simulink model "Test"  (R2018b)
settings: Solver=VariableStepAuto  StartTime=0.0  StopTime=10.0  RelTol=1e-3
undefined symbols (not defined in the file or in its folder): ExpectedOutputs, Inputs, sigbuilder_block, TestCase, TestInps, TestIters
libraries: fillib x3, library x2
(part 3 of 7)

== stateflow chart Test/ XOR ==
  settings: stateMachineType=SIMPLIFIED_MACHINE
  state Init
    fb_select = 1;
    dataInA = 67108864;
    dataInB = 67108864;
    fb_control.enableIn = logical(1);
    fb_control.enableOut = logical(1);
    fb_control.enableResult = logical(1);
    fb_control.reset = logical(0);
  state step_1
    fb_select = 5;
    dataInA = int32(Inputs(TestInps,1));
    dataInB = int32(Inputs(TestInps,1));
    fb_control.enableIn = logical(1);
    fb_control.enableOut = logical(0);
    fb_control.enableResult = logical(0);
    fb_control.reset = logical(0);
    verify(fb_functions_out.numInputs ==4);
    verify(fb_functions_out.numOutputs ==2);
    verify(fb_functions_out.fb_error_code ==256);
    verify(fb_functions_out.dataOut == 0);
    verify(fb_functions_out.state_error == 0);
    verify(fb_functions_out.executed == 1);
  state step_2
    fb_select = 5;
    dataInA = 67108864;
    dataInB = 67108864;
    fb_control.enableIn = logical(0);
    fb_control.enableOut = logical(0);
    fb_control.enableResult = logical(0);
    fb_control.reset = logical(0);
    verify(fb_functions_out.numInputs ==4);
    verify(fb_functions_out.numOutputs ==2);
    verify(fb_functions_out.fb_error_code == 256);
    verify(fb_functions_out.dataOut == 0);
    verify(fb_functions_out.state_error == 0);
    verify(fb_functions_out.executed == 1);
  state step_3
    fb_select = 5;
    dataInA = int32(Inputs(TestInps,2));
    dataInB = int32(Inputs(TestInps,2));
    fb_control.enableIn = logical(1);
    fb_control.enableOut = logical(0);
    fb_control.enableResult = logical(0);
    fb_control.reset = logical(0);
    verify(fb_functions_out.numInputs ==4);
    verify(fb_functions_out.numOutputs ==2);
    verify(fb_functions_out.fb_error_code == 256);
    verify(fb_functions_out.dataOut == 0);
    verify(fb_functions_out.state_error == 0);
    verify(fb_functions_out.executed == 1);
  state step_12
    fb_select = 5;
    dataInA = 0;
    dataInB = 0;
    fb_control.enableIn = logical(0);
    fb_control.enableOut = logical(0);
    fb_control.enableResult = logical(0);
    fb_control.reset = logical(0);
    verify(fb_functions_out.numInputs ==4);
    verify(fb_functions_out.numOutputs ==2);
    verify(fb_functions_out.fb_error_code == 256);
    verify(fb_functions_out.dataOut == 0);
    verify(fb_functions_out.state_error == 0);
    verify(fb_functions_out.executed == 1);
  state step_15
    fb_select = 5;
    dataInA = int32(Inputs(TestInps,3));
    dataInB = int32(Inputs(TestInps,3));
    fb_control.enableIn = logical(1);
    fb_control.enableOut = logical(0);
    fb_control.enableResult = logical(0);
    fb_control.reset = logical(0);
    verify(fb_functions_out.numInputs ==4);
    verify(fb_functions_out.numOutputs ==2);
    verify(fb_functions_out.fb_error_code == 256);
    verify(fb_functions_out.dataOut == 0);
    verify(fb_functions_out.state_error == 0);
    verify(fb_functions_out.executed == 1);
  state step_16
    fb_select = 5;
    dataInA = 67108864;
    dataInB = 67108864;
    fb_control.enableIn = logical(0);
    fb_control.enableOut = logical(0);
    fb_control.enableResult = logical(0);
    fb_control.reset = logical(0);
    verify(fb_functions_out.numInputs ==4);
    verify(fb_functions_out.numOutputs ==2);
    verify(fb_functions_out.fb_error_code == 256);
    verify(fb_functions_out.dataOut == 0);
    verify(fb_functions_out.state_error == 0);
    verify(fb_functions_out.executed == 1);
  state step_13
    fb_select = 5;
    dataInA = int32(Inputs(TestInps,4));
    dataInB = int32(Inputs(TestInps,4));
    fb_control.enableIn = logical(1);
    fb_control.enableOut = logical(0);
    fb_control.enableResult = logical(0);
    fb_control.reset = logical(0);
    verify(fb_functions_out.numInputs ==4);
    verify(fb_functions_out.numOutputs ==2);
    verify(fb_functions_out.fb_error_code == 256);
    verify(fb_functions_out.dataOut == 0);
    verify(fb_functions_out.state_error == 0);
    verify(fb_functions_out.executed == 1);
  state step_14
    fb_select = 5;
    dataInA = 0;
    dataInB = 0;
    fb_control.enableIn = logical(0);
    fb_control.enableOut = logical(0);
    fb_control.enableResult = logical(0);
    fb_control.reset = logical(0);
    verify(fb_functions_out.numInputs ==4);
    verify(fb_functions_out.numOutputs ==2);
    verify(fb_functions_out.fb_error_code == 256);
    verify(fb_functions_out.dataOut == 0);
    verify(fb_functions_out.state_error == 0);
    verify(fb_functions_out.executed == 1);
  state step_4
    fb_select = 5;
    dataInA = 0;
    dataInB = 0;
    fb_control.enableIn = logical(0);
    fb_control.enableOut = logical(0);
    fb_control.enableResult = logical(1);
    fb_control.reset =logical(0);
    verify(fb_functions_out.numInputs ==4);
    verify(fb_functions_out.numOutputs ==2);
    verify(fb_functions_out.fb_error_code == uint32(ExpectedOutputs(TestInps,3)));
    verify(fb_functions_out.dataOut == 0);
    verify(fb_functions_out.state_error == 0);
    verify(fb_functions_out.executed == 1);
  state step_5
    fb_select = 5;
    dataInA = 674;
    dataInB = 673;
    fb_control.enableIn = logical(0);
    fb_control.enableOut = logical(0);
    fb_control.enableResult = logical(0);
    fb_control.reset = logical(0);
    verify(fb_functions_out.numInputs == 4);
    verify(fb_functions_out.numOutputs ==2);
    verify(fb_functions_out.fb_error_code == uint32(ExpectedOutputs(TestInps,3)));
    verify(fb_functions_out.dataOut == 0);
    verify(fb_functions_out.state_error == 0);
    verify(fb_functions_out.executed == 1);
  state step_6
    fb_select = 5;
    dataInA = 674;
    dataInB = 673;
    fb_control.enableIn = logical(0);
    fb_control.enableOut = logical(1);
    fb_control.enableResult = logical(0);
    fb_control.reset = logical(0);
    verify(fb_functions_out.numInputs ==4);
    verify(fb_functions_out.numOutputs ==2);
    verify(fb_functions_out.fb_error_code == uint32(ExpectedOutputs(TestInps,3)));
    verify(fb_functions_out.dataOut == int32(ExpectedOutputs(TestInps,1)));
    ActualOutputs(TestInps,3)= int32(fb_functions_out.fb_error_code);
    ActualOutputs(TestInps,1)= int32(fb_functions_out.dataOut);
    verify(fb_functions_out.state_error == 0);
    verify(fb_functions_out.executed == 1);
  state step_7
    fb_select = 5;
    dataInA = 674;
    dataInB = 673;
    fb_control.enableIn = logical(0);
    fb_control.enableOut = logical(0);
    fb_control.enableResult = logical(0);
    fb_control.reset = logical(0);
    verify(fb_functions_out.numInputs ==4);
    verify(fb_functions_out.numOutputs ==2);
    verify(fb_functions_out.fb_error_code == uint32(ExpectedOutputs(TestInps,3)));
    verify(fb_functions_out.dataOut == int32(ExpectedOutputs(TestInps,1)));
    verify(fb_functions_out.state_error == 0);
    verify(fb_functions_out.executed == 1);
  state step_8
    fb_select = 5;
    dataInA = 674;
    dataInB = 673;
    fb_control.enableIn = logical(0);
    fb_control.enableOut = logical(1);
    fb_control.enableResult = logical(0);
    fb_control.reset = logical(0);
    verify(fb_functions_out.numInputs ==4);
    verify(fb_functions_out.numOutputs ==2);
    verify(fb_functions_out.fb_error_code == uint32(ExpectedOutputs(TestInps,3)));
    verify(fb_functions_out.dataOut == int32(ExpectedOutputs(TestInps,2)));
    ActualOutputs(TestInps,2)= int32(fb_functions_out.dataOut);
    verify(fb_functions_out.state_error == 0);
    verify(fb_functions_out.executed == 1);
  state step_9
    fb_select = 5;
    dataInA = 674;
    dataInB = 673;
    fb_control.enableIn = logical(0);
    fb_control.enableOut = logical(0);
    fb_control.enableResult = logical(0);
    fb_control.reset = logical(0);
    verify(fb_functions_out.numInputs ==4);
    verify(fb_functions_out.numOutputs ==2);
    verify(fb_functions_out.fb_error_code == uint32(ExpectedOutputs(TestInps,3)));
    verify(fb_functions_out.dataOut == int32(ExpectedOutputs(TestInps,2)));
    verify(fb_functions_out.state_error == 0);
    verify(fb_functions_out.executed == 1);
  state step_10
    fb_select = 5;
    dataInA = 674;
    dataInB = 673;
    fb_control.enableIn = logical(0);
    fb_control.enableOut = logical(0);
    fb_control.enableResult = logical(0);
    fb_control.reset = logical(0);
    verify(fb_functions_out.numInputs ==4);
    verify(fb_functions_out.numOutputs == 2);
    verify(fb_functions_out.fb_error_code == uint32(ExpectedOutputs(TestInps,3)));
    verify(fb_functions_out.dataOut == 0);
    verify(fb_functions_out.state_error == 0);
    verify(fb_functions_out.executed == 1);
  state step_11
    fb_select = 5;
    dataInA = 67108864;
    dataInB = 142606336;
    fb_control.enableIn = logical(1);
    fb_control.enableOut = logical(0);
    fb_control.enableResult = logical(0);
    fb_control.reset = logical(0);
    verify(fb_functions_out.numInputs ==4);
    verify(fb_functions_out.numOutputs ==2);
    verify(fb_functions_out.fb_error_code ==256);
    verify(fb_functions_out.dataOut == 0);
    verify(fb_functions_out.state_error == 0);
    verify(fb_functions_out.executed == 1);
  state step_17
    fb_select = 5;
    dataInA = 18000;
    dataInB = 18000;
    fb_control.enableIn = logical(1);
    fb_control.enableOut = logical(0);
    fb_control.enableResult = logical(0);
    fb_control.reset = logical(0);
    verify(fb_functions_out.numInputs ==4);
    verify(fb_functions_out.numOutputs ==2);
    verify(fb_functions_out.fb_error_code ==256);
    verify(fb_functions_out.dataOut == 0);
    verify(fb_functions_out.state_error == 0);
    verify(fb_functions_out.executed == 1);
  state step_18
    fb_select = 5;
    dataInA = 67108864;
    dataInB = 67108864;
    fb_control.enableIn = logical(1);
    fb_control.enableOut = logical(0);
    fb_control.enableResult = logical(0);
    fb_control.reset = logical(0);
    verify(fb_functions_out.numInputs ==4);
    verify(fb_functions_out.numOutputs ==2);
    verify(fb_functions_out.fb_error_code ==256);
    verify(fb_functions_out.dataOut == 0);
    verify(fb_functions_out.state_error == 1);
    verify(fb_functions_out.executed == 1);
  state step_19
    fb_select = 5;
    dataInA = 15000;
    dataInB = 15000;
    fb_control.enableIn = logical(1);
    fb_control.enableOut = logical(0);
    fb_control.enableResult = logical(0);
    fb_control.reset = logical(0);
    verify(fb_functions_out.numInputs ==4);
    verify(fb_functions_out.numOutputs ==2);
    verify(fb_functions_out.fb_error_code ==256);
    verify(fb_functions_out.dataOut == 0);
    verify(fb_functions_out.state_error == 1);
    verify(fb_functions_out.executed == 1);
  state step_20
    fb_select = 5;
    dataInA = 15000;
    dataInB = 15000;
    fb_control.enableIn = logical(0);
    fb_control.enableOut = logical(0);
    fb_control.enableResult = logical(0);
    fb_control.reset = logical(0);
    verify(fb_functions_out.numInputs ==4);
    verify(fb_functions_out.numOutputs ==2);
    verify(fb_functions_out.fb_error_code ==256);
    verify(fb_functions_out.dataOut == 0);
    verify(fb_functions_out.state_error == 1);
    verify(fb_functions_out.executed == 1);
  state step_21
    fb_select = 5;
    dataInA = 15000;
    dataInB = 15000;
    fb_control.enableIn = logical(0);
    fb_control.enableOut = logical(0);
    fb_control.enableResult = logical(1);
    fb_control.reset = logical(0);
    verify(fb_functions_out.numInputs ==4);
    verify(fb_functions_out.numOutputs ==2);
    verify(fb_functions_out.fb_error_code ==256);
    verify(fb_functions_out.dataOut == 0);
    verify(fb_functions_out.state_error == 1);
    verify(fb_functions_out.executed == 1);
  state step_22
    fb_select = 5;
    dataInA = 15000;
    dataInB = 15000;
    fb_control.enableIn = logical(0);
    fb_control.enableOut = logical(0);
    fb_control.enableResult = logical(0);
    fb_control.reset = logical(0);
    verify(fb_functions_out.numInputs ==4);
    verify(fb_functions_out.numOutputs ==2);
    verify(fb_functions_out.fb_error_code ==256);
    verify(fb_functions_out.dataOut == 0);
    verify(fb_functions_out.state_error == 1);
    verify(fb_functions_out.executed == 1);
  state step_23
    fb_select = 5;
    dataInA = 15000;
    dataInB = 15000;
    fb_control.enableIn = logical(0);
    fb_control.enableOut = logical(1);
    fb_control.enableResult = logical(0);
    fb_control.reset = logical(0);
    verify(fb_functions_out.numInputs ==4);
    verify(fb_functions_out.numOutputs ==2);
    verify(fb_functions_out.fb_error_code ==256);
    %verify(fb_functions_out.dataOut ==16777216);
    verify(fb_functions_out.dataOut ==67108864);
    verify(fb_functions_out.state_error == 1);
    verify(fb_functions_out.executed == 1);
  state step_24
    fb_select = 5;
    dataInA = 15000;
    dataInB = 15000;
    fb_control.enableIn = logical(0);
    fb_control.enableOut = logical(1);
    fb_control.enableResult = logical(0);
    fb_control.reset = logical(0);
    verify(fb_functions_out.numInputs ==4);
    verify(fb_functions_out.numOutputs ==2);
    verify(fb_functions_out.fb_error_code ==256);
    %verify(fb_functions_out.dataOut == 16777216);
    verify(fb_functions_out.dataOut ==67108864);
    verify(fb_functions_out.state_error == 1);
    verify(fb_functions_out.executed == 1);
  state step_25
    fb_select = 5;
    dataInA = 15000;
    dataInB = 15000;
    fb_control.enableIn = logical(0);
    fb_control.enableOut = logical(0);
    fb_control.enableResult = logical(0);
    fb_control.reset = logical(0);
    verify(fb_functions_out.numInputs ==4);
    verify(fb_functions_out.numOutputs ==2);
    verify(fb_functions_out.fb_error_code ==256);
    verify(fb_functions_out.dataOut ==0);
    verify(fb_functions_out.state_error == 1);
    verify(fb_functions_out.executed == 1);
  state step_26
    fb_select = 5;
    dataInA = 16777216;
    dataInB = 16777216;
    fb_control.enableIn = logical(1);
    fb_control.enableOut = logical(0);
    fb_control.enableResult = logical(0);
    fb_control.reset = logical(0);
    verify(fb_functions_out.numInputs ==4);
    verify(fb_functions_out.numOutputs ==2);
    verify(fb_functions_out.fb_error_code ==256);
    verify(fb_functions_out.dataOut ==0);
    verify(fb_functions_out.state_error == 0);
    verify(fb_functions_out.executed == 1);
  state step_27
    fb_select = 5;
    dataInA = 0;
    dataInB = 1;
    fb_control.enableIn = logical(1);
    fb_control.enableOut = logical(0);
    fb_control.enableResult = logical(0);
    fb_control.reset = logical(0);
    verify(fb_functions_out.numInputs ==4);
    verify(fb_functions_out.numOutputs ==2);
    verify(fb_functions_out.fb_error_code ==256);
    verify(fb_functions_out.dataOut ==0);
    verify(fb_functions_out.state_error == 0);
    verify(fb_functions_out.executed == 1);
  state step_28
    fb_select = 5;
    dataInA = 16777216;
    dataInB = 16777216;
    fb_control.enableIn = logical(1);
    fb_control.enableOut = logical(0);
    fb_control.enableResult = logical(0);
    fb_control.reset = logical(0);
    verify(fb_functions_out.numInputs ==4);
    verify(fb_functions_out.numOutputs ==2);
    verify(fb_functions_out.fb_error_code ==256);
    verify(fb_functions_out.dataOut ==0);
    verify(fb_functions_out.state_error == 0);
    verify(fb_functions_out.executed == 1);
  state step_29
    fb_select = 5;
    dataInA = 1;
    dataInB = 1;
    fb_control.enableIn = logical(1);
    fb_control.enableOut = logical(0);
    fb_control.enableResult = logical(0);
    fb_control.reset = logical(0);
    verify(fb_functions_out.numInputs ==4);
    verify(fb_functions_out.numOutputs ==2);
    verify(fb_functions_out.fb_error_code ==256);
    verify(fb_functions_out.dataOut ==0);
    verify(fb_functions_out.state_error == 1);
    verify(fb_functions_out.executed == 1);
  state step_35
    fb_select = 5;
    dataInA = 1;
    dataInB = 1;
    fb_control.enableIn = logical(0);
    fb_control.enableOut = logical(0);
    fb_control.enableResult = logical(0);
    fb_control.reset = logical(0);
    verify(fb_functions_out.numInputs ==4);
    verify(fb_functions_out.numOutputs ==2);
    verify(fb_functions_out.fb_error_code ==256);
    verify(fb_functions_out.dataOut ==0);
    verify(fb_functions_out.state_error == 1);
    verify(fb_functions_out.executed == 1);
  state step_30
    fb_select = 5;
    dataInA = 1;
    dataInB = 1;
    fb_control.enableIn = logical(0);
    fb_control.enableOut = logical(0);
    fb_control.enableResult = logical(1);
    fb_control.reset = logical(0);
    verify(fb_functions_out.numInputs ==4);
    verify(fb_functions_out.numOutputs ==2);
    verify(fb_functions_out.fb_error_code ==0);
    verify(fb_functions_out.dataOut ==0);
    verify(fb_functions_out.state_error == 1);
    verify(fb_functions_out.executed == 1);
  state step_31
    fb_select = 5;
    dataInA = 1;
    dataInB = 1;
    fb_control.enableIn = logical(0);
    fb_control.enableOut = logical(0);
    fb_control.enableResult = logical(0);
    fb_control.reset = logical(0);
    verify(fb_functions_out.numInputs ==4);
    verify(fb_functions_out.numOutputs ==2);
    verify(fb_functions_out.fb_error_code ==0);
    verify(fb_functions_out.dataOut ==0);
    verify(fb_functions_out.state_error == 1);
    verify(fb_functions_out.executed == 1);
  state step_32
    fb_select = 5;
    dataInA = 1;
    dataInB = 1;
    fb_control.enableIn = logical(0);
    fb_control.enableOut = logical(1);
    fb_control.enableResult = logical(0);
    fb_control.reset = logical(0);
    verify(fb_functions_out.numInputs ==4);
    verify(fb_functions_out.numOutputs ==2);
    verify(fb_functions_out.fb_error_code ==0);
    verify(fb_functions_out.dataOut ==16777216);
    verify(fb_functions_out.state_error == 1);
    verify(fb_functions_out.executed == 1);
  state step_33
    fb_select = 5;
    dataInA = 1;
    dataInB = 1;
    fb_control.enableIn = logical(0);
    fb_control.enableOut = logical(0);
    fb_control.enableResult = logical(0);
    fb_control.reset = logical(0);
    verify(fb_functions_out.numInputs ==4);
    verify(fb_functions_out.numOutputs ==2);
    verify(fb_functions_out.fb_error_code ==0);
    verify(fb_functions_out.dataOut == 16777216);
    verify(fb_functions_out.state_error == 1);
    verify(fb_functions_out.executed == 1);
  state step_34
    fb_select = 5;
    dataInA = 1;
    dataInB = 1;
    fb_control.enableIn = logical(0);
    fb_control.enableOut = logical(1);
    fb_control.enableResult = logical(0);
    fb_control.reset = logical(0);
    verify(fb_functions_out.numInputs ==4);
    verify(fb_functions_out.numOutputs ==2);
    verify(fb_functions_out.fb_error_code ==0);
    verify(fb_functions_out.dataOut == 1);
    verify(fb_functions_out.state_error == 1);
    verify(fb_functions_out.executed == 1);
  state End_Test
  (default) -> Init
  Init -> (junction 246) [order 2] : [after(1,tick) && (TestCase == 2)
      | ]
  (junction 246) -> (junction 126)
  Init -> (junction 248) [order 3] : [after(1,tick) && (TestCase == 3)
      | ]
  (junction 248) -> (junction 221)
  Init -> step_1 [order 1] : [after(1,tick) && (TestCase == 1)
      | ]
  step_1 -> step_2 : [after(1,tick)
      | ]
  step_2 -> step_3 : [after(1,tick)
      | ]
  step_3 -> step_12 : [after(1,tick)
      | ]
  step_12 -> step_15 : [after(1,tick)
      | ]
  step_15 -> step_16 : [after(1,tick)
      | ]
  step_16 -> step_13 : [after(1,tick)
      | ]
  step_13 -> step_14 : [after(1,tick)
      | ]
  step_14 -> step_4 : [after(1,tick)
      | ]
  step_4 -> step_5 : [after(1,tick)
      | ]
  step_5 -> step_6 : [after(1,tick)
      | ]
  step_6 -> step_7 : [after(1,tick)
      | ]
  step_7 -> step_8 : [after(1,tick)
      | ]
  step_8 -> step_9 : [after(1,tick)
      | ]
  step_9 -> step_10 : [after(1,tick)
      | ]
  step_10 -> (junction 122) : [after(1,tick)
      | ]
  (junction 122) -> (junction 169)
  (junction 126) -> step_11
  step_11 -> step_17 : [after(1,tick)
      | ]
  step_17 -> step_18 : [after(1,tick)
      | ]
  step_18 -> step_19 : [after(1,tick)
      | ]
  step_19 -> step_20 : [after(1,tick)
      | ]
  step_20 -> step_21 : [after(1,tick)
      | ]
  step_21 -> step_22 : [after(1,tick)
      | ]
  step_22 -> step_23 : [after(1,tick)
      | ]
  step_23 -> step_24 : [after(1,tick)
      | ]
  step_24 -> step_25 : [after(1,tick)
      | ]
  step_25 -> (junction 169) : [after(1,tick)
      | ]
  (junction 169) -> (junction 120)
  (junction 221) -> step_26
  step_26 -> step_27 : [after(1,tick)
      | ]
  step_27 -> step_28 : [after(1,tick)
      | ]
  step_28 -> step_29 : [after(1,tick)
      | ]
  step_29 -> step_35 : [after(1,tick)
      | ]
  step_35 -> step_30 : [after(1,tick)
      | ]
  step_30 -> step_31 : [after(1,tick)
      | ]
  step_31 -> step_32 : [after(1,tick)
      | ]
  step_32 -> step_33 : [after(1,tick)
      | ]
  step_33 -> step_34 : [after(1,tick)
      | ]
  step_34 -> End_Test : [after(1,tick)
      | ]
  (junction 120) -> End_Test
  data: fb_select output double size=[1]; fb_control output Bus: fb_control size=[1]; dataInA output int32 size=[1]; dataInB output int32 size=[1]; fb_functions_out input Bus: fb_functions_out; TestCase parameter uint8; ExpectedOutputs parameter int32 size=[TestIters, 3]; Inputs parameter int32 size=[TestIters, 4]; ActualOutputs data_store_memory; TestInps parameter uint8

== stateflow chart Test/Test Sequence ==
  settings: stateMachineType=SIMPLIFIED_MACHINE
  state Init
    fb_select = 1;
    dataInA = 67108864;
    dataInB = 67108864;
    fb_control.enableIn = logical(1);
    fb_control.enableOut = logical(1);
    fb_control.enableResult = logical(1);
    fb_control.reset = logical(0);
  state step_1
    fb_select = 2;
    dataInA = int32(Inputs(TestInps,1));
    dataInB = int32(Inputs(TestInps,1));
    fb_control.enableIn = logical(1);
    fb_control.enableOut = logical(0);
    fb_control.enableResult = logical(0);
    fb_control.reset = logical(0);
    verify(fb_functions_out.numInputs ==4);
    verify(fb_functions_out.numOutputs ==2);
    verify(fb_functions_out.fb_error_code ==256);
    verify(fb_functions_out.dataOut == 0);
    verify(fb_functions_out.state_error == 0);
    verify(fb_functions_out.executed == 1);
  state step_2
    fb_select = 2;
    dataInA = 67108864;
    dataInB = 67108864;
    fb_control.enableIn = logical(0);
    fb_control.enableOut = logical(0);
    fb_control.enableResult = logical(0);
    fb_control.reset = logical(0);
    verify(fb_functions_out.numInputs ==4);
    verify(fb_functions_out.numOutputs ==2);
    verify(fb_functions_out.fb_error_code == 256);
    verify(fb_functions_out.dataOut == 0);
    verify(fb_functions_out.state_error == 0);
    verify(fb_functions_out.executed == 1);
  state step_3
    fb_select = 2;
    dataInA = int32(Inputs(TestInps,2));
    dataInB = int32(Inputs(TestInps,2));
    fb_control.enableIn = logical(1);
    fb_control.enableOut = logical(0);
    fb_control.enableResult = logical(0);
    fb_control.reset = logical(0);
    verify(fb_functions_out.numInputs ==4);
    verify(fb_functions_out.numOutputs ==2);
    verify(fb_functions_out.fb_error_code == 256);
    verify(fb_functions_out.dataOut == 0);
    verify(fb_functions_out.state_error == 0);
    verify(fb_functions_out.executed == 1);
  state step_12
    fb_select = 2;
    dataInA = 0;
    dataInB = 0;
    fb_control.enableIn = logical(0);
    fb_control.enableOut = logical(0);
    fb_control.enableResult = logical(0);
    fb_control.reset = logical(0);
    verify(fb_functions_out.numInputs ==4);
    verify(fb_functions_out.numOutputs ==2);
    verify(fb_functions_out.fb_error_code == 256);
    verify(fb_functions_out.dataOut == 0);
    verify(fb_functions_out.state_error == 0);
    verify(fb_functions_out.executed == 1);
  state step_15
    fb_select = 2;
    dataInA = int32(Inputs(TestInps,3));
    dataInB = int32(Inputs(TestInps,3));
    fb_control.enableIn = logical(1);
    fb_control.enableOut = logical(0);
    fb_control.enableResult = logical(0);
    fb_control.reset = logical(0);
    verify(fb_functions_out.numInputs ==4);
    verify(fb_functions_out.numOutputs ==2);
    verify(fb_functions_out.fb_error_code == 256);
    verify(fb_functions_out.dataOut == 0);
    verify(fb_functions_out.state_error == 0);
    verify(fb_functions_out.executed == 1);
  state step_16
    fb_select = 2;
    dataInA = 67108864;
    dataInB = 67108864;
    fb_control.enableIn = logical(0);
    fb_control.enableOut = logical(0);
    fb_control.enableResult = logical(0);
    fb_control.reset = logical(0);
    verify(fb_functions_out.numInputs ==4);
    verify(fb_functions_out.numOutputs ==2);
    verify(fb_functions_out.fb_error_code == 256);
    verify(fb_functions_out.dataOut == 0);
    verify(fb_functions_out.state_error == 0);
    verify(fb_functions_out.executed == 1);
  state step_13
    fb_select = 2;
    dataInA = int32(Inputs(TestInps,4));
    dataInB = int32(Inputs(TestInps,4));
    fb_control.enableIn = logical(1);
    fb_control.enableOut = logical(0);
    fb_control.enableResult = logical(0);
    fb_control.reset = logical(0);
    verify(fb_functions_out.numInputs ==4);
    verify(fb_functions_out.numOutputs ==2);
    verify(fb_functions_out.fb_error_code == 256);
    verify(fb_functions_out.dataOut == 0);
    verify(fb_functions_out.state_error == 0);
    verify(fb_functions_out.executed == 1);
  state step_14
    fb_select = 2;
    dataInA = 0;
    dataInB = 0;
    fb_control.enableIn = logical(0);
    fb_control.enableOut = logical(0);
    fb_control.enableResult = logical(0);
    fb_control.reset = logical(0);
    verify(fb_functions_out.numInputs ==4);
    verify(fb_functions_out.numOutputs ==2);
    verify(fb_functions_out.fb_error_code == 256);
    verify(fb_functions_out.dataOut == 0);
    verify(fb_functions_out.state_error == 0);
    verify(fb_functions_out.executed == 1);
  state step_4
    fb_select = 2;
    dataInA = 0;
    dataInB = 0;
    fb_control.enableIn = logical(0);
    fb_control.enableOut = logical(0);
    fb_control.enableResult = logical(1);
    fb_control.reset =logical(0);
    verify(fb_functions_out.numInputs ==4);
    verify(fb_functions_out.numOutputs ==2);
    verify(fb_functions_out.fb_error_code == uint32(ExpectedOutputs(TestInps,3)));
    verify(fb_functions_out.dataOut == 0);
    verify(fb_functions_out.state_error == 0);
    verify(fb_functions_out.executed == 1);
  state step_5
    fb_select = 2;
    dataInA = 674;
    dataInB = 673;
    fb_control.enableIn = logical(0);
    fb_control.enableOut = logical(0);
    fb_control.enableResult = logical(0);
    fb_control.reset = logical(0);
    verify(fb_functions_out.numInputs == 4);
    verify(fb_functions_out.numOutputs ==2);
    verify(fb_functions_out.fb_error_code == uint32(ExpectedOutputs(TestInps,3)));
    verify(fb_functions_out.dataOut == 0);
    verify(fb_functions_out.state_error == 0);
    verify(fb_functions_out.executed == 1);
  state step_6
    fb_select = 2;
    dataInA = 674;
    dataInB = 673;
    fb_control.enableIn = logical(0);
    fb_control.enableOut = logical(1);
    fb_control.enableResult = logical(0);
    fb_control.reset = logical(0);
    verify(fb_functions_out.numInputs ==4);
    verify(fb_functions_out.numOutputs ==2);
    verify(fb_functions_out.fb_error_code == uint32(ExpectedOutputs(TestInps,3)));
    verify(fb_functions_out.dataOut == int32(ExpectedOutputs(TestInps,1)));
    ActualOutputs(TestInps,3)= int32(fb_functions_out.fb_error_code);
    ActualOutputs(TestInps,1)= int32(fb_functions_out.dataOut);
    verify(fb_functions_out.state_error == 0);
    verify(fb_functions_out.executed == 1);
  state step_7
    fb_select = 2;
    dataInA = 674;
    dataInB = 673;
    fb_control.enableIn = logical(0);
    fb_control.enableOut = logical(0);
    fb_control.enableResult = logical(0);
    fb_control.reset = logical(0);
    verify(fb_functions_out.numInputs ==4);
    verify(fb_functions_out.numOutputs ==2);
    verify(fb_functions_out.fb_error_code == uint32(ExpectedOutputs(TestInps,3)));
    verify(fb_functions_out.dataOut == int32(ExpectedOutputs(TestInps,1)));
    verify(fb_functions_out.state_error == 0);
    verify(fb_functions_out.executed == 1);
  state step_8
    fb_select = 2;
    dataInA = 674;
    dataInB = 673;
    fb_control.enableIn = logical(0);
    fb_control.enableOut = logical(1);
    fb_control.enableResult = logical(0);
    fb_control.reset = logical(0);
    verify(fb_functions_out.numInputs ==4);
    verify(fb_functions_out.numOutputs ==2);
    verify(fb_functions_out.fb_error_code == uint32(ExpectedOutputs(TestInps,3)));
    verify(fb_functions_out.dataOut == int32(ExpectedOutputs(TestInps,2)));
    ActualOutputs(TestInps,2)= int32(fb_functions_out.dataOut);
    verify(fb_functions_out.state_error == 0);
    verify(fb_functions_out.executed == 1);
  state step_9
    fb_select = 2;
    dataInA = 674;
    dataInB = 673;
    fb_control.enableIn = logical(0);
    fb_control.enableOut = logical(0);
    fb_control.enableResult = logical(0);
    fb_control.reset = logical(0);
    verify(fb_functions_out.numInputs ==4);
    verify(fb_functions_out.numOutputs ==2);
    verify(fb_functions_out.fb_error_code == uint32(ExpectedOutputs(TestInps,3)));
    verify(fb_functions_out.dataOut == int32(ExpectedOutputs(TestInps,2)));
    verify(fb_functions_out.state_error == 0);
    verify(fb_functions_out.executed == 1);
  state step_10
    fb_select = 2;
    dataInA = 674;
    dataInB = 673;
    fb_control.enableIn = logical(0);
    fb_control.enableOut = logical(0);
    fb_control.enableResult = logical(0);
    fb_control.reset = logical(0);
    verify(fb_functions_out.numInputs ==4);
    verify(fb_functions_out.numOutputs == 2);
    verify(fb_functions_out.fb_error_code == uint32(ExpectedOutputs(TestInps,3)));
    verify(fb_functions_out.dataOut == 0);
    verify(fb_functions_out.state_error == 0);
    verify(fb_functions_out.executed == 1);
  state step_11
    fb_select = 2;
    dataInA = 67108864;
    dataInB = 142606336;
    fb_control.enableIn = logical(1);
    fb_control.enableOut = logical(0);
    fb_control.enableResult = logical(0);
    fb_control.reset = logical(0);
    verify(fb_functions_out.numInputs ==4);
    verify(fb_functions_out.numOutputs ==2);
    verify(fb_functions_out.fb_error_code ==256);
    verify(fb_functions_out.dataOut == 0);
    verify(fb_functions_out.state_error == 0);
    verify(fb_functions_out.executed == 1);
  state step_17
    fb_select = 2;
    dataInA = 18000;
    dataInB = 18000;
    fb_control.enableIn = logical(1);
    fb_control.enableOut = logical(0);
    fb_control.enableResult = logical(0);
    fb_control.reset = logical(0);
    verify(fb_functions_out.numInputs ==4);
    verify(fb_functions_out.numOutputs ==2);
    verify(fb_functions_out.fb_error_code ==256);
    verify(fb_functions_out.dataOut == 0);
    verify(fb_functions_out.state_error == 0);
    verify(fb_functions_out.executed == 1);
  state step_18
    fb_select = 2;
    dataInA = 67108864;
    dataInB = 67108864;
    fb_control.enableIn = logical(1);
    fb_control.enableOut = logical(0);
    fb_control.enableResult = logical(0);
    fb_control.reset = logical(0);
    verify(fb_functions_out.numInputs ==4);
    verify(fb_functions_out.numOutputs ==2);
    verify(fb_functions_out.fb_error_code ==256);
    verify(fb_functions_out.dataOut == 0);
    verify(fb_functions_out.state_error == 1);
    verify(fb_functions_out.executed == 1);
  state step_19
    fb_select = 2;
    dataInA = 15000;
    dataInB = 15000;
    fb_control.enableIn = logical(1);
    fb_control.enableOut = logical(0);
    fb_control.enableResult = logical(0);
    fb_control.reset = logical(0);
    verify(fb_functions_out.numInputs ==4);
    verify(fb_functions_out.numOutputs ==2);
    verify(fb_functions_out.fb_error_code ==256);
    verify(fb_functions_out.dataOut == 0);
    verify(fb_functions_out.state_error == 1);
    verify(fb_functions_out.executed == 1);
  state step_20
    fb_select = 2;
    dataInA = 15000;
    dataInB = 15000;
    fb_control.enableIn = logical(0);
    fb_control.enableOut = logical(0);
    fb_control.enableResult = logical(0);
    fb_control.reset = logical(0);
    verify(fb_functions_out.numInputs ==4);
    verify(fb_functions_out.numOutputs ==2);
    verify(fb_functions_out.fb_error_code ==256);
    verify(fb_functions_out.dataOut == 0);
    verify(fb_functions_out.state_error == 1);
    verify(fb_functions_out.executed == 1);
  state step_21
    fb_select = 2;
    dataInA = 15000;
    dataInB = 15000;
    fb_control.enableIn = logical(0);
    fb_control.enableOut = logical(0);
    fb_control.enableResult = logical(1);
    fb_control.reset = logical(0);
    verify(fb_functions_out.numInputs ==4);
    verify(fb_functions_out.numOutputs ==2);
    verify(fb_functions_out.fb_error_code ==256);
    verify(fb_functions_out.dataOut == 0);
    verify(fb_functions_out.state_error == 1);
    verify(fb_functions_out.executed == 1);
  state step_22
    fb_select = 2;
    dataInA = 15000;
    dataInB = 15000;
    fb_control.enableIn = logical(0);
    fb_control.enableOut = logical(0);
    fb_control.enableResult = logical(0);
    fb_control.reset = logical(0);
    verify(fb_functions_out.numInputs ==4);
    verify(fb_functions_out.numOutputs ==2);
    verify(fb_functions_out.fb_error_code ==256);
    verify(fb_functions_out.dataOut == 0);
    verify(fb_functions_out.state_error == 1);
    verify(fb_functions_out.executed == 1);
  state step_23
    fb_select = 2;
    dataInA = 15000;
    dataInB = 15000;
    fb_control.enableIn = logical(0);
    fb_control.enableOut = logical(1);
    fb_control.enableResult = logical(0);
    fb_control.reset = logical(0);
    verify(fb_functions_out.numInputs ==4);
    verify(fb_functions_out.numOutputs ==2);
    verify(fb_functions_out.fb_error_code ==256);
    %verify(fb_functions_out.dataOut ==16777216);
    verify(fb_functions_out.dataOut ==67108864);
    verify(fb_functions_out.state_error == 1);
    verify(fb_functions_out.executed == 1);
  state step_24
    fb_select = 2;
    dataInA = 15000;
    dataInB = 15000;
    fb_control.enableIn = logical(0);
    fb_control.enableOut = logical(1);
    fb_control.enableResult = logical(0);
    fb_control.reset = logical(0);
    verify(fb_functions_out.numInputs ==4);
    verify(fb_functions_out.numOutputs ==2);
    verify(fb_functions_out.fb_error_code ==256);
    %verify(fb_functions_out.dataOut == 16777216);
    verify(fb_functions_out.dataOut ==67108864);
    verify(fb_functions_out.state_error == 1);
    verify(fb_functions_out.executed == 1);
  state step_25
    fb_select = 2;
    dataInA = 15000;
    dataInB = 15000;
    fb_control.enableIn = logical(0);
    fb_control.enableOut = logical(0);
    fb_control.enableResult = logical(0);
    fb_control.reset = logical(0);
    verify(fb_functions_out.numInputs ==4);
    verify(fb_functions_out.numOutputs ==2);
    verify(fb_functions_out.fb_error_code ==256);
    verify(fb_functions_out.dataOut ==1);
    verify(fb_functions_out.state_error == 1);
    verify(fb_functions_out.executed == 1);
  state step_26
    fb_select = 2;
    dataInA = 16777216;
    dataInB = 16777216;
    fb_control.enableIn = logical(1);
    fb_control.enableOut = logical(0);
    fb_control.enableResult = logical(0);
    fb_control.reset = logical(0);
    verify(fb_functions_out.numInputs ==4);
    verify(fb_functions_out.numOutputs ==2);
    verify(fb_functions_out.fb_error_code ==256);
    verify(fb_functions_out.dataOut ==0);
    verify(fb_functions_out.state_error == 0);
    verify(fb_functions_out.executed == 1);
  state step_27
    fb_select = 2;
    dataInA = 0;
    dataInB = 1;
    fb_control.enableIn = logical(1);
    fb_control.enableOut = logical(0);
    fb_control.enableResult = logical(0);
    fb_control.reset = logical(0);
    verify(fb_functions_out.numInputs ==4);
    verify(fb_functions_out.numOutputs ==2);
    verify(fb_functions_out.fb_error_code ==256);
    verify(fb_functions_out.dataOut ==0);
    verify(fb_functions_out.state_error == 0);
    verify(fb_functions_out.executed == 1);
  state step_28
    fb_select = 2;
    dataInA = 16777216;
    dataInB = 16777216;
    fb_control.enableIn = logical(1);
    fb_control.enableOut = logical(0);
    fb_control.enableResult = logical(0);
    fb_control.reset = logical(0);
    verify(fb_functions_out.numInputs ==4);
    verify(fb_functions_out.numOutputs ==2);
    verify(fb_functions_out.fb_error_code ==256);
    verify(fb_functions_out.dataOut ==0);
    verify(fb_functions_out.state_error == 0);
    verify(fb_functions_out.executed == 1);
  state step_29
    fb_select = 2;
    dataInA = 1;
    dataInB = 1;
    fb_control.enableIn = logical(1);
    fb_control.enableOut = logical(0);
    fb_control.enableResult = logical(0);
    fb_control.reset = logical(0);
    verify(fb_functions_out.numInputs ==4);
    verify(fb_functions_out.numOutputs ==2);
    verify(fb_functions_out.fb_error_code ==256);
    verify(fb_functions_out.dataOut ==0);
    verify(fb_functions_out.state_error == 1);
    verify(fb_functions_out.executed == 1);
  state step_35
    fb_select = 2;
    dataInA = 1;
    dataInB = 1;
    fb_control.enableIn = logical(0);
    fb_control.enableOut = logical(0);
    fb_control.enableResult = logical(0);
    fb_control.reset = logical(0);
    verify(fb_functions_out.numInputs ==4);
    verify(fb_functions_out.numOutputs ==2);
    verify(fb_functions_out.fb_error_code ==256);
    verify(fb_functions_out.dataOut ==0);
    verify(fb_functions_out.state_error == 1);
    verify(fb_functions_out.executed == 1);
  state step_30
    fb_select = 2;
    dataInA = 1;
    dataInB = 1;
    fb_control.enableIn = logical(0);
    fb_control.enableOut = logical(0);
    fb_control.enableResult = logical(1);
    fb_control.reset = logical(0);
    verify(fb_functions_out.numInputs ==4);
    verify(fb_functions_out.numOutputs ==2);
    verify(fb_functions_out.fb_error_code ==0);
    verify(fb_functions_out.dataOut ==0);
    verify(fb_functions_out.state_error == 1);
    verify(fb_functions_out.executed == 1);
  state step_31
    fb_select = 2;
    dataInA = 1;
    dataInB = 1;
    fb_control.enableIn = logical(0);
    fb_control.enableOut = logical(0);
    fb_control.enableResult = logical(0);
    fb_control.reset = logical(0);
    verify(fb_functions_out.numInputs ==4);
    verify(fb_functions_out.numOutputs ==2);
    verify(fb_functions_out.fb_error_code ==0);
    verify(fb_functions_out.dataOut ==0);
    verify(fb_functions_out.state_error == 1);
    verify(fb_functions_out.executed == 1);
  state step_32
    fb_select = 2;
    dataInA = 1;
    dataInB = 1;
    fb_control.enableIn = logical(0);
    fb_control.enableOut = logical(1);
    fb_control.enableResult = logical(0);
    fb_control.reset = logical(0);
    verify(fb_functions_out.numInputs ==4);
    verify(fb_functions_out.numOutputs ==2);
    verify(fb_functions_out.fb_error_code ==0);
    verify(fb_functions_out.dataOut ==16777216);
    verify(fb_functions_out.state_error == 1);
    verify(fb_functions_out.executed == 1);
  state step_33
    fb_select = 2;
    dataInA = 1;
    dataInB = 1;
    fb_control.enableIn = logical(0);
    fb_control.enableOut = logical(0);
    fb_control.enableResult = logical(0);
    fb_control.reset = logical(0);
    verify(fb_functions_out.numInputs ==4);
    verify(fb_functions_out.numOutputs ==2);
    verify(fb_functions_out.fb_error_code ==0);
    verify(fb_functions_out.dataOut == 16777216);
    verify(fb_functions_out.state_error == 1);
    verify(fb_functions_out.executed == 1);
  state step_34
    fb_select = 2;
    dataInA = 1;
    dataInB = 1;
    fb_control.enableIn = logical(0);
    fb_control.enableOut = logical(1);
    fb_control.enableResult = logical(0);
    fb_control.reset = logical(0);
    verify(fb_functions_out.numInputs ==4);
    verify(fb_functions_out.numOutputs ==2);
    verify(fb_functions_out.fb_error_code ==0);
    verify(fb_functions_out.dataOut == 0);
    verify(fb_functions_out.state_error == 1);
    verify(fb_functions_out.executed == 1);
  state End_Test
  (default) -> Init
  Init -> (junction 239) [order 2] : [after(1,tick) && (TestCase == 2)
      | ]
  (junction 239) -> (junction 126)
  Init -> (junction 243) [order 3] : [after(1,tick) && (TestCase == 3)
      | ]
  (junction 243) -> (junction 221)
  Init -> step_1 [order 1] : [after(1,tick) && (TestCase == 1)
      | ]
  step_1 -> step_2 : [after(1,tick)
      | ]
  step_2 -> step_3 : [after(1,tick)
      | ]
  step_3 -> step_12 : [after(1,tick)
      | ]
  step_12 -> step_15 : [after(1,tick)
      | ]
  step_15 -> step_16 : [after(1,tick)
      | ]
  step_16 -> step_13 : [after(1,tick)
      | ]
  step_13 -> step_14 : [after(1,tick)
      | ]
  step_14 -> step_4 : [after(1,tick)
      | ]
  step_4 -> step_5 : [after(1,tick)
      | ]
  step_5 -> step_6 : [after(1,tick)
      | ]
  step_6 -> step_7 : [after(1,tick)
      | ]
  step_7 -> step_8 : [after(1,tick)
      | ]
  step_8 -> step_9 : [after(1,tick)
      | ]
  step_9 -> step_10 : [after(1,tick)
      | ]
  step_10 -> (junction 122) : [after(1,tick)
      | ]
  (junction 122) -> (junction 169)
  (junction 126) -> step_11
  step_11 -> step_17 : [after(1,tick)
      | ]
  step_17 -> step_18 : [after(1,tick)
      | ]
  step_18 -> step_19 : [after(1,tick)
      | ]
  step_19 -> step_20 : [after(1,tick)
      | ]
  step_20 -> step_21 : [after(1,tick)
      | ]
  step_21 -> step_22 : [after(1,tick)
      | ]
  step_22 -> step_23 : [after(1,tick)
      | ]
  step_23 -> step_24 : [after(1,tick)
      | ]
  step_24 -> step_25 : [after(1,tick)
      | ]
  step_25 -> (junction 169) : [after(1,tick)
      | ]
  (junction 169) -> (junction 120)
  (junction 221) -> step_26
  step_26 -> step_27 : [after(1,tick)
      | ]
  step_27 -> step_28 : [after(1,tick)
      | ]
  step_28 -> step_29 : [after(1,tick)
      | ]
  step_29 -> step_35 : [after(1,tick)
      | ]
  step_35 -> step_30 : [after(1,tick)
      | ]
  step_30 -> step_31 : [after(1,tick)
      | ]
  step_31 -> step_32 : [after(1,tick)
      | ]
  step_32 -> step_33 : [after(1,tick)
      | ]
  step_33 -> step_34 : [after(1,tick)
      | ]
  step_34 -> End_Test : [after(1,tick)
      | ]
  (junction 120) -> End_Test
  data: fb_select output double size=[1]; fb_control output Bus: fb_control size=[1]; dataInA output int32 size=[1]; dataInB output int32 size=[1]; fb_functions_out input Bus: fb_functions_out; TestCase parameter uint8; ExpectedOutputs parameter int32 size=[TestIters, 3]; Inputs parameter int32 size=[TestIters, 4]; ActualOutputs data_store_memory; TestInps parameter uint8
